simulink library "dspddes3"  (Simulink 5.0)
libraries: dsparch4 x7
settings Model: RequirementInfo=9  Creator=dshpak  LastModifiedBy=mkhan  TargetHWChar=2  TargetHWWordLengths=8,16,32,32

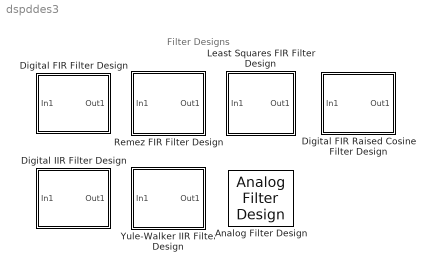
== system dspddes3 ==
  note: Filter Designs
  Analog Filter Design : dsparch4/Analog Filter Design  method=Butterworth  filttype=Lowpass  N=8  Wlo=30  Whi=80  Rp=2  Rs=40
  Digital FIR Filter Design : Subsystem  mask(Digital FIR Filter Design){filttype=Lowpass, N=22, Wlo=0.4, Whi=0.6, W0=[.2 .5 .8], g0=1, W1=[0 .2 .3 .6 .8 1], gains=[1 .5 0 0 1 .5], wintype=Hamming, Rs=10, Kbeta=5}
      mask prompts: filttype "Filter type:"; N "Filter order:"; Wlo "Cutoff frequency (0 to 1):"; Whi "Upper cutoff frequency:"; W0 "Cutoff frequency vector (0 < f < 1):"; g0 "Gain in the first band:"; W1 "Frequency vector (including 0 and 1):"; gains "Gains at these frequencies:"; wintype "Window type:"; Rs "Stopband attenuation in dB:"; Kbeta "Beta:"
      mask help: Implements various window-based FIR filter designs using the Signal Processing Toolbox's "fir1" and "fir2" filter design commands. The gain at each "cutoff frequency" is the average of the gains in the adjacent bands (usually 0.5).
      mask init:
      | [b,h,w,str]=dspblkfir2('design',filttype,N,Wlo,Whi,W0,g0,W1,gains,wintype,Rs, Kbeta);
      mask Help: web(dspbhelp);
      mask StyleString: popup(Lowpass|Highpass|Bandpass|Bandstop|Multiband|Arbitrary Shape (fir2)),edit,edit,edit,edit,popup(0|1),edit,edit,popup(Bartlett|Blackman|Boxcar|Chebyshev|Hamming|Hann|Hanning|Kaiser|Triangular),edit,edit
      mask CallbackString: dspblkfir2||||||||dspblkfir2||
      mask Display: plot(w,h); text(.05,.9,str);
  Digital FIR Raised Cosine Filter Design : Subsystem  mask(Digital FIR Raised Cosine Filter Design){filter_order=63, upper_cutoff_freq=0.5, enable_sqrt_design=on, rolloff_type=Rolloff factor, transition_bw=0.4, rolloff_factor=0.6, window_type=Boxcar, Rs=5, Kbeta=10, InitCond=0}
      mask prompts: filter_order "Filter order:"; upper_cutoff_freq "Upper cutoff frequency (0 to 1):"; enable_sqrt_design "Square-root raised cosine filter"; rolloff_type "Design method:"; transition_bw "Transition bandwidth (0 < Df < 1):"; rolloff_factor "Rolloff factor (0 to 1):"; window_type "Window type:"; Rs "Stopband attenuation in dB:"; Kbeta "Beta:"; InitCond "Initial conditions:"
      mask help: Linear phase digital FIR lowpass raised cosine filter.
      mask init:
      | [str,h,w,b]= dspblkfirrcos2('design',filter_order,upper_cutoff_freq,rolloff_type,transition_bw,rolloff_factor, window_type, Rs, enable_sqrt_design, Kbeta);
      mask Help: web(dspbhelp);
      mask StyleString: edit,edit,checkbox,popup(Transition bandwidth|Rolloff factor),edit,edit,popup(Bartlett|Blackman|Boxcar|Chebyshev|Hamming|Hann|Hanning|Kaiser|Triangular),edit,edit,edit
      mask CallbackString: |||dspblkfirrcos2|||dspblkfirrcos2|||
      mask Display:
      | plot(w,h);
      | text(.05,.9,str);
  Digital IIR Filter Design : Subsystem  mask(Digital IIR Filter Design){method=Butterworth, filttype=Lowpass, N=4, Wlo=0.4, Whi=0.6, Rp=2, Rs=20}
      mask prompts: method "Design method:"; filttype "Filter type:"; N "Filter order:"; Wlo "Passband edge frequency (0 to 1):"; Whi "Should not be visible!"; Rp "Passband ripple in dB:"; Rs "Stopband attenuation in dB:"
      mask help: Design one of several standard IIR filters, implemented in direct form.
      mask init:
      | [b,a,h,w,str] = dspblkiir2('design',method,filttype,N,...
      |                                               Wlo,Whi,Rp,Rs);
      mask Help: web(dspbhelp);
      mask StyleString: popup(Butterworth|Chebyshev I|Chebyshev II|Elliptic),popup(Lowpass|Highpass|Bandpass|Bandstop),edit,edit,edit,edit,edit
      mask CallbackString: dspblkiir2|dspblkiir2|||||
      mask Display: plot(w,h); text(.05,.9,str);
  Least Squares FIR Filter Design : Subsystem  mask(Least Squares FIR Filter Design){filttype=Multiband, N=12, F=[0 0.3 0.6 1], A=[0 0 1 1], W=[1 1]}
      mask prompts: filttype "Filter type:"; N "Filter order:"; F "Band-edge frequency vector (including 0 and 1):"; A "Gains at these frequencies:"; W "Weights (one per band):"
      mask help: Least-squares linear phase FIR filter.
      mask init:
      | [b,h,w,str] = dspblkfirls2('design',filttype,N,F,A,W);
      mask Help: web(dspbhelp);
      mask StyleString: popup(Multiband|Hilbert Transformer|Differentiator),edit,edit,edit,edit
      mask Display: plot(w,h); text(.05,.9,str);
  Remez FIR Filter Design : Subsystem  mask(Remez FIR Filter Design){filttype=Multiband, F=[0 0.4 0.5 1], A=[1 1 0 0], W=[1 1], N=23}
      mask prompts: filttype "Filter type:"; F "Band-edge frequency vector (including 0 and 1):"; A "Gains at these frequencies:"; W "Weights (one per band):"; N "Filter order:"
      mask help: Parks-McClellan linear phase FIR filter.
      mask init:
      | [b,h,w,str] = dspblkremez2('design', filttype,N,F,A,W);
      mask Help: web(dspbhelp);
      mask StyleString: popup(Multiband|Hilbert Transformer|Differentiator),edit,edit,edit,edit
      mask Display: plot(w,h); text(.05,.9,str);
  Yule-Walker IIR Filter Design : Subsystem  mask(Yule-Walker IIR Filter Design){N=8, F=[0 .4 .6 1], A=[1 1 0 0]}
      mask prompts: N "Filter order:"; F "Band-edge frequency vector (including 0 and 1):"; A "Magnitudes at these frequencies:"
      mask help: Yule-Walker IIR filter design.
      mask init:
      | [b,a,h,w,str] = dspblkyule2('design', N,F,A);
      mask Help: web(dspbhelp);
      mask Display: plot(w,h); text(.05,.9,str);

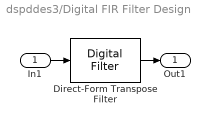
== system dspddes3/Digital FIR Filter Design ==
  In1 : Inport
  Direct-Form Transpose Filter : dsparch4/Digital Filter  TypePopup=FIR (all zeros)  IIRFiltStruct=Direct form II transposed  AllPoleFiltStruct=Direct form  FIRFiltStruct=Direct form transposed  CoeffSource=Specify via dialog  NumCoeffs=b  DenCoeffs=1  BiQuadCoeffs=[1 0.3 0.4 1 0.1 0.2]  LatticeCoeffs=[0.2 0.4]  denIgnore=on  FiltPerSampPopup=One filter per frame  IC=0  ICnum=0  ICden=0
  Out1 : Outport  InitialOutput=0
  wires:
  In1/1 -> Direct-Form Transpose Filter/1
  Direct-Form Transpose Filter/1 -> Out1/1

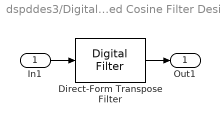
== system dspddes3/Digital FIR Raised Cosine Filter Design ==
  In1 : Inport
  Direct-Form Transpose Filter : dsparch4/Digital Filter  TypePopup=FIR (all zeros)  IIRFiltStruct=Direct form II transposed  AllPoleFiltStruct=Direct form  FIRFiltStruct=Direct form transposed  CoeffSource=Specify via dialog  NumCoeffs=b  DenCoeffs=1  BiQuadCoeffs=[1 0.3 0.4 1 0.1 0.2]  LatticeCoeffs=[0.2 0.4]  denIgnore=on  FiltPerSampPopup=One filter per frame  IC=InitCond  ICnum=0  ICden=0
  Out1 : Outport
  wires:
  In1/1 -> Direct-Form Transpose Filter/1
  Direct-Form Transpose Filter/1 -> Out1/1

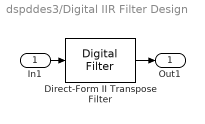
== system dspddes3/Digital IIR Filter Design ==
  In1 : Inport
  Direct-Form II Transpose Filter : dsparch4/Digital Filter  TypePopup=IIR (poles & zeros)  IIRFiltStruct=Direct form II transposed  AllPoleFiltStruct=Direct form  FIRFiltStruct=Direct form transposed  CoeffSource=Specify via dialog  NumCoeffs=b  DenCoeffs=a  BiQuadCoeffs=[1 0.3 0.4 1 0.1 0.2]  LatticeCoeffs=[0.2 0.4]  denIgnore=on  FiltPerSampPopup=One filter per frame  IC=0  ICnum=0  ICden=0
  Out1 : Outport  InitialOutput=0
  wires:
  In1/1 -> Direct-Form II Transpose Filter/1
  Direct-Form II Transpose Filter/1 -> Out1/1

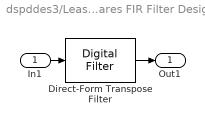
== system dspddes3/Least Squares FIR Filter Design ==
  In1 : Inport
  Direct-Form Transpose Filter : dsparch4/Digital Filter  TypePopup=FIR (all zeros)  IIRFiltStruct=Direct form II transposed  AllPoleFiltStruct=Direct form  FIRFiltStruct=Direct form transposed  CoeffSource=Specify via dialog  NumCoeffs=b  DenCoeffs=1  BiQuadCoeffs=[1 0.3 0.4 1 0.1 0.2]  LatticeCoeffs=[0.2 0.4]  denIgnore=on  FiltPerSampPopup=One filter per frame  IC=0  ICnum=0  ICden=0
  Out1 : Outport  InitialOutput=0
  wires:
  In1/1 -> Direct-Form Transpose Filter/1
  Direct-Form Transpose Filter/1 -> Out1/1

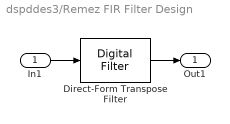
== system dspddes3/Remez FIR Filter Design ==
  In1 : Inport
  Direct-Form Transpose Filter : dsparch4/Digital Filter  TypePopup=FIR (all zeros)  IIRFiltStruct=Direct form II transposed  AllPoleFiltStruct=Direct form  FIRFiltStruct=Direct form transposed  CoeffSource=Specify via dialog  NumCoeffs=b  DenCoeffs=1  BiQuadCoeffs=[1 0.3 0.4 1 0.1 0.2]  LatticeCoeffs=[0.2 0.4]  denIgnore=on  FiltPerSampPopup=One filter per frame  IC=0  ICnum=0  ICden=0
  Out1 : Outport  InitialOutput=0
  wires:
  Direct-Form Transpose Filter/1 -> Out1/1
  In1/1 -> Direct-Form Transpose Filter/1

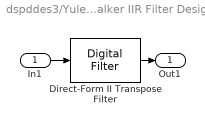
== system dspddes3/Yule-Walker IIR Filter Design ==
  In1 : Inport
  Direct-Form II Transpose Filter : dsparch4/Digital Filter  TypePopup=IIR (poles & zeros)  IIRFiltStruct=Direct form II transposed  AllPoleFiltStruct=Direct form  FIRFiltStruct=Direct form transposed  CoeffSource=Specify via dialog  NumCoeffs=b  DenCoeffs=a  BiQuadCoeffs=[1 0.3 0.4 1 0.1 0.2]  LatticeCoeffs=[0.2 0.4]  denIgnore=on  FiltPerSampPopup=One filter per frame  IC=0  ICnum=0  ICden=0
  Out1 : Outport  InitialOutput=0
  wires:
  In1/1 -> Direct-Form II Transpose Filter/1
  Direct-Form II Transpose Filter/1 -> Out1/1
